simulink model "LQGsim"  (R2017a)
settings: Solver=ode3  StartTime=0.0  StopTime=100.0  FixedStep=0.001  RelTol=1e-3  EnableMultiTasking=on
values from neighbouring files (symbols this model uses):
  K = lqr(A,B,Q,R)    [LQGexample.m]
libraries: cstblocks x3
settings Model: Creator=ian  LastModifiedBy=ian
settings DataIOCC: LimitDataPoints=on  SaveFormat=Array
settings OptimizationCC: ExpressionDepthLimit=2147483647  LifeSpan=inf
settings DebuggingCC: UnderspecifiedInitializationDetection=Classic  MergeDetectMultiDrivingBlocksExec=none  SolverPrmCheckMsg=warning  StateNameClashWarn=warning  SFUnexpectedBacktrackingDiag=warning  SFNoUnconditionalDefaultTransitionDiag=warning  SFExecutionAtInitializationDiag=none
settings HardwareCC: ProdBitPerPointer=32  ProdBitPerSizeT=32  ProdBitPerPtrDiffT=32  ProdLargestAtomicFloat=None  ProdIntDivRoundTo=Undefined  ProdEndianess=Unspecified  ProdWordSize=32  ProdHWDeviceType=32-bit Generic
settings ModelReferenceCC: PropagateSignalLabelsOutOfModel=off
settings GRTTargetCC: TargetLangStandard=C89/C90 (ANSI)  GeneratePreprocessorConditionals=Disable all
settings ConfigComp: CovMetricSettings=dw  CovHtmlReporting=on  CovSaveCumulativeToWorkspaceVar=on  CovSaveSingleToWorkspaceVar=on  CovExternalEMLEnable=off

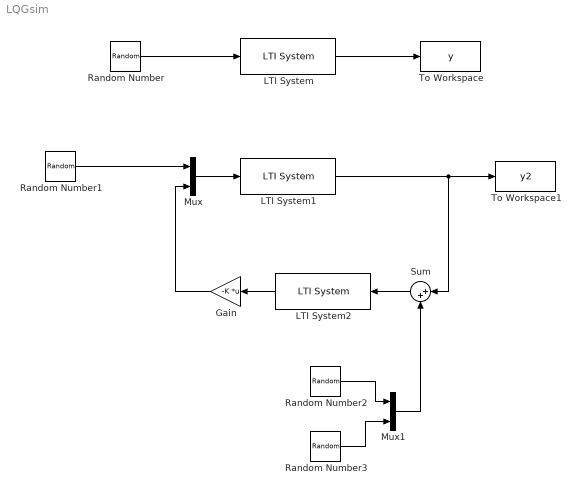
== system LQGsim ==
  Gain : Gain  Gain=-K  Multiplication=Matrix(K*u)
  LTI System : cstblocks/LTI System  sys=sys  IC=[]
  LTI System1 : cstblocks/LTI System  sys=sys2  IC=[]
  LTI System2 : cstblocks/LTI System  sys=kalmanfilt  IC=[]
  Mux : Mux  Inputs=2
  Mux1 : Mux  Inputs=2
  Random Number : RandomNumber  Seed=floor(100*rand)  SampleTime=0.001
  Random Number1 : RandomNumber  Seed=floor(100*rand)  SampleTime=0.001
  Random Number2 : RandomNumber  Variance=1e-6  Seed=floor(100*rand)  SampleTime=0.001
  Random Number3 : RandomNumber  Variance=1e-6  Seed=floor(100*rand)  SampleTime=0.001
  Sum : Sum  Inputs=|++
  To Workspace : ToWorkspace  VariableName=y  SampleTime=-1
  To Workspace1 : ToWorkspace  VariableName=y2  SampleTime=-1
  wires:
  LTI System/1 -> To Workspace/1
  Random Number/1 -> LTI System/1
  LTI System1/1 -> Sum/1, To Workspace1/1
  LTI System2/1 -> Gain/1
  Random Number1/1 -> Mux/1
  Gain/1 -> Mux/2
  Mux/1 -> LTI System1/1
  Sum/1 -> LTI System2/1
  Random Number2/1 -> Mux1/1
  Random Number3/1 -> Mux1/2
  Mux1/1 -> Sum/2
